simulink model "com_simulink"  (R2026a)
settings: Solver=VariableStepAuto  StopTime=Inf
libraries: instrumentseriallib x2
settings Model: Creator=Claudio  LastModifiedBy=Dante P

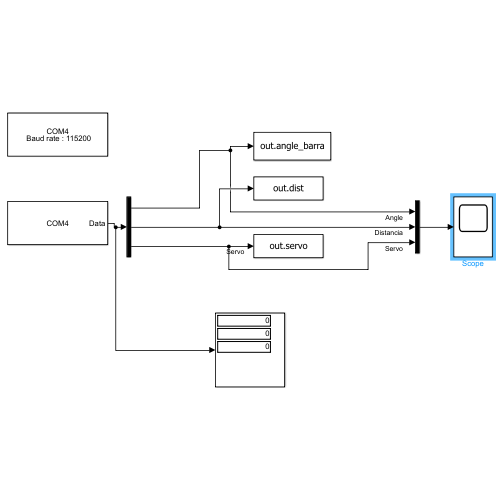
[thumbnail: Simulink's stored preview of the top-level diagram]
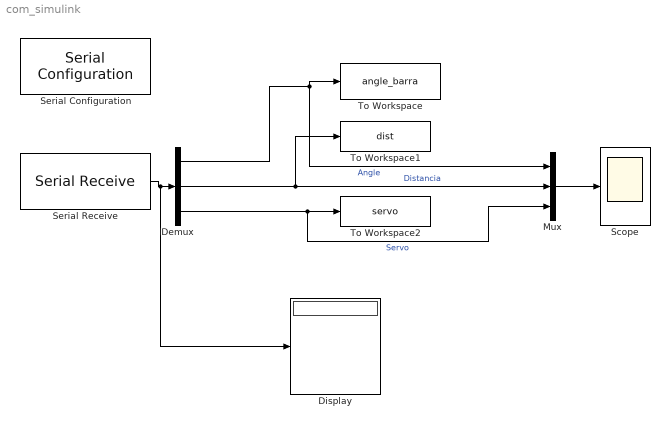
== system com_simulink ==
  Demux : Demux  Outputs=3
  Display : Display
  Mux : Mux  Inputs=3
  Scope : Scope
      settings: TimeSpan=60  ActiveDisplayYMinimum=-1.9454486018782617  ActiveDisplayYMaximum=8.4937052880648576
  Serial Configuration : instrumentseriallib/Serial Configuration  Priority=-200000  PortSel=COM4  Port=COM4  ComPort=COM4  BaudRate=115200  DataBits=8  Parity=none  StopBits=1  ByteOrder=big-endian  FlowControl=none  Timeout=10  SimulateUsing=Interpreted execution  BlockInModel=on  aMode=1
  Serial Receive : instrumentseriallib/Serial Receive  Priority=1  PortSel=COM4  Port=COM4  ComPort=COM4  DataType=single  SaveDataType=uint8  ToggleHeader=on  Header="[ 97   98   99  100 ]"  ToggleDataSize=on  DataSize=[3 1]  ToggleTerminator=off  Terminator=<none>  CustomTerminator=[]  InputFormat=Column major  EnableBlockingMode=on  ActionDataUnavailable=Output last received value  ActionWhenDataUnavailable=Output last received value  CustomValue=0  SampleTime=0.02  SimulateUsing=Interpreted execution  BlockInModel=on  aMode=1  LibraryInUse=instrumentlib
  To Workspace : ToWorkspace  VariableName=angle_barra  SampleTime=-1
      settings: Save2DSignal=2-D array (concatenate along first dimension)
  To Workspace1 : ToWorkspace  VariableName=dist  SampleTime=-1
      settings: Save2DSignal=2-D array (concatenate along first dimension)
  To Workspace2 : ToWorkspace  VariableName=servo  SampleTime=-1
      settings: Save2DSignal=2-D array (concatenate along first dimension)
  wires:
  Demux/2 -> To Workspace1/1, Mux/2  "Distancia"
  Demux/1 -> To Workspace/1, Mux/1  "Angle"
  Serial Receive/1 -> Display/1, Demux/1
  Demux/3 -> To Workspace2/1, Mux/3  "Servo"
  Mux/1 -> Scope/1
